simulink model "MCU_FOC_MAIN"  (R2024b)
settings: configuration reference "MODEL_CONFIG_PARENT" (kept outside this file)
settings Model: DataDictionary=MCU_FOC_MAIN_DD.sldd  EnableAccessToBaseWorkspace=off  Creator=415  LastModifiedBy=415
settings ConfigSetRef: SourceName=MODEL_CONFIG_PARENT

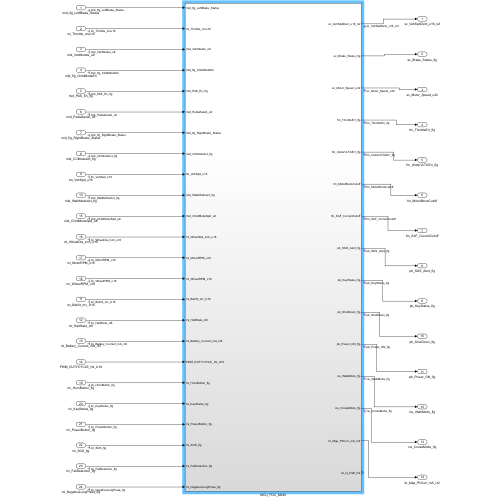
[thumbnail: Simulink's stored preview of the top-level diagram]
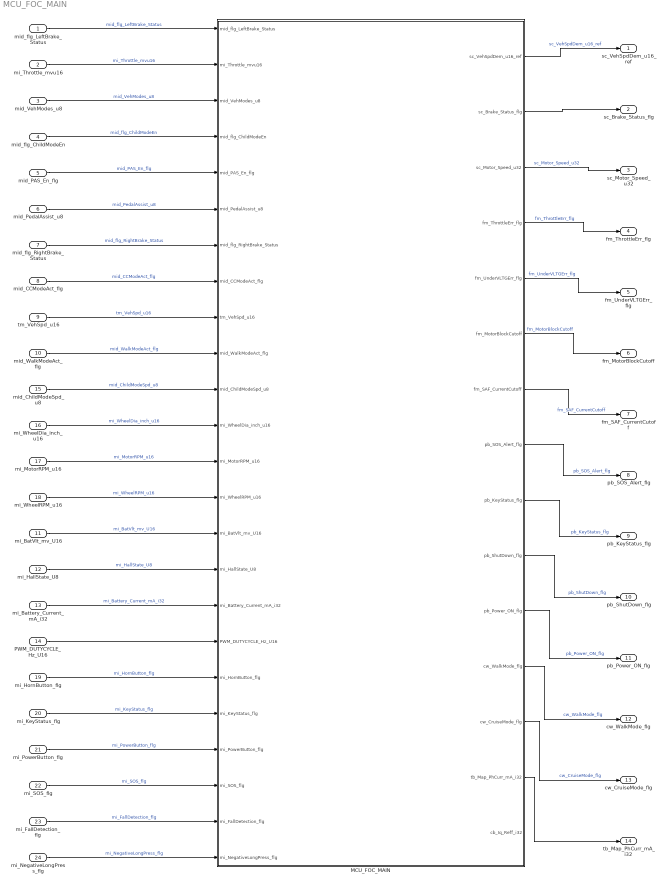
== system MCU_FOC_MAIN ==
  mid_flg_LeftBrake_Status : Inport
  mi_Throttle_mvu16 : Inport  Port=2
  mid_VehModes_u8 : Inport  Port=3
  mid_flg_ChildModeEn : Inport  Port=4
  mid_PAS_En_flg : Inport  Port=5
  mid_PedalAssist_u8 : Inport  Port=6
  mid_flg_RightBrake_Status : Inport  Port=7
  mid_CCModeAct_flg : Inport  Port=8
  tm_VehSpd_u16 : Inport  Port=9
  mid_WalkModeAct_flg : Inport  Port=10
  mi_BatVlt_mv_U16 : Inport  Port=11
  mi_HallState_U8 : Inport  Port=12
  mi_Battery_Current_mA_i32 : Inport  Port=13
  PWM_DUTYCYCLE_Hz_U16 : Inport  Port=14
  mid_ChildModeSpd_u8 : Inport  Port=15
  mi_WheelDia_inch_u16 : Inport  Port=16
  mi_MotorRPM_u16 : Inport  Port=17
  mi_WheelRPM_u16 : Inport  Port=18
  mi_HornButton_flg : Inport  Port=19
  mi_KeyStatus_flg : Inport  Port=20
  mi_PowerButton_flg : Inport  Port=21
  mi_SOS_flg : Inport  Port=22
  mi_FallDetection_flg : Inport  Port=23
  mi_NegativeLongPress_flg : Inport  Port=24
  MCU_FOC_MAIN : Subsystem
  sc_VehSpdDem_u16_ref : Outport
  sc_Brake_Status_flg : Outport  Port=2
  sc_Motor_Speed_u32 : Outport  Port=3
  fm_ThrottleErr_flg : Outport  Port=4
  fm_UnderVLTGErr_flg : Outport  Port=5
  fm_MotorBlockCutoff : Outport  Port=6
  fm_SAF_CurrentCutoff : Outport  Port=7
  pb_SOS_Alert_flg : Outport  Port=8
  pb_KeyStatus_flg : Outport  Port=9
  pb_ShutDown_flg : Outport  Port=10
  pb_Power_ON_flg : Outport  Port=11
  cw_WalkMode_flg : Outport  Port=12
  cw_CruiseMode_flg : Outport  Port=13
  tb_Map_PhCurr_mA_i32 : Outport  Port=14
  wires:
  mid_PedalAssist_u8/1 -> MCU_FOC_MAIN/6(mid_PedalAssist_u8)  "mid_PedalAssist_u8"
  mid_flg_RightBrake_Status/1 -> MCU_FOC_MAIN/7(mid_flg_RightBrake_Status)  "mid_flg_RightBrake_Status"
  mid_flg_LeftBrake_Status/1 -> MCU_FOC_MAIN/1(mid_flg_LeftBrake_Status)  "mid_flg_LeftBrake_Status"
  MCU_FOC_MAIN/13(cw_CruiseMode_flg) -> cw_CruiseMode_flg/1  "cw_CruiseMode_flg"
  mi_Throttle_mvu16/1 -> MCU_FOC_MAIN/2(mi_Throttle_mvu16)  "mi_Throttle_mvu16"
  mid_flg_ChildModeEn/1 -> MCU_FOC_MAIN/4(mid_flg_ChildModeEn)  "mid_flg_ChildModeEn"
  mi_NegativeLongPress_flg/1 -> MCU_FOC_MAIN/24(mi_NegativeLongPress_flg)  "mi_NegativeLongPress_flg"
  mid_VehModes_u8/1 -> MCU_FOC_MAIN/3(mid_VehModes_u8)  "mid_VehModes_u8"
  mi_BatVlt_mv_U16/1 -> MCU_FOC_MAIN/15(mi_BatVlt_mv_U16)  "mi_BatVlt_mv_U16"
  mid_PAS_En_flg/1 -> MCU_FOC_MAIN/5(mid_PAS_En_flg)  "mid_PAS_En_flg"
  mid_CCModeAct_flg/1 -> MCU_FOC_MAIN/8(mid_CCModeAct_flg)  "mid_CCModeAct_flg"
  MCU_FOC_MAIN/7(fm_SAF_CurrentCutoff) -> fm_SAF_CurrentCutoff/1  "fm_SAF_CurrentCutoff"
  tm_VehSpd_u16/1 -> MCU_FOC_MAIN/9(tm_VehSpd_u16)  "tm_VehSpd_u16"
  mid_WalkModeAct_flg/1 -> MCU_FOC_MAIN/10(mid_WalkModeAct_flg)  "mid_WalkModeAct_flg"
  mid_ChildModeSpd_u8/1 -> MCU_FOC_MAIN/11(mid_ChildModeSpd_u8)  "mid_ChildModeSpd_u8"
  mi_HallState_U8/1 -> MCU_FOC_MAIN/16(mi_HallState_U8)  "mi_HallState_U8"
  mi_WheelDia_inch_u16/1 -> MCU_FOC_MAIN/12(mi_WheelDia_inch_u16)  "mi_WheelDia_inch_u16"
  mi_Battery_Current_mA_i32/1 -> MCU_FOC_MAIN/17(mi_Battery_Current_mA_i32)  "mi_Battery_Current_mA_i32"
  mi_MotorRPM_u16/1 -> MCU_FOC_MAIN/13(mi_MotorRPM_u16)  "mi_MotorRPM_u16"
  MCU_FOC_MAIN/3(sc_Motor_Speed_u32) -> sc_Motor_Speed_u32/1  "sc_Motor_Speed_u32"
  PWM_DUTYCYCLE_Hz_U16/1 -> MCU_FOC_MAIN/18(PWM_DUTYCYCLE_Hz_U16)
  mi_WheelRPM_u16/1 -> MCU_FOC_MAIN/14(mi_WheelRPM_u16)  "mi_WheelRPM_u16"
  MCU_FOC_MAIN/12(cw_WalkMode_flg) -> cw_WalkMode_flg/1  "cw_WalkMode_flg"
  mi_HornButton_flg/1 -> MCU_FOC_MAIN/19(mi_HornButton_flg)  "mi_HornButton_flg"
  mi_KeyStatus_flg/1 -> MCU_FOC_MAIN/20(mi_KeyStatus_flg)  "mi_KeyStatus_flg"
  mi_PowerButton_flg/1 -> MCU_FOC_MAIN/21(mi_PowerButton_flg)  "mi_PowerButton_flg"
  mi_SOS_flg/1 -> MCU_FOC_MAIN/22(mi_SOS_flg)  "mi_SOS_flg"
  mi_FallDetection_flg/1 -> MCU_FOC_MAIN/23(mi_FallDetection_flg)  "mi_FallDetection_flg"
  MCU_FOC_MAIN/1(sc_VehSpdDem_u16_ref) -> sc_VehSpdDem_u16_ref/1  "sc_VehSpdDem_u16_ref"
  MCU_FOC_MAIN/2(sc_Brake_Status_flg) -> sc_Brake_Status_flg/1
  MCU_FOC_MAIN/4(fm_ThrottleErr_flg) -> fm_ThrottleErr_flg/1  "fm_ThrottleErr_flg"
  MCU_FOC_MAIN/8(pb_SOS_Alert_flg) -> pb_SOS_Alert_flg/1  "pb_SOS_Alert_flg"
  MCU_FOC_MAIN/5(fm_UnderVLTGErr_flg) -> fm_UnderVLTGErr_flg/1  "fm_UnderVLTGErr_flg"
  MCU_FOC_MAIN/6(fm_MotorBlockCutoff) -> fm_MotorBlockCutoff/1  "fm_MotorBlockCutoff"
  MCU_FOC_MAIN/9(pb_KeyStatus_flg) -> pb_KeyStatus_flg/1  "pb_KeyStatus_flg"
  MCU_FOC_MAIN/10(pb_ShutDown_flg) -> pb_ShutDown_flg/1  "pb_ShutDown_flg"
  MCU_FOC_MAIN/11(pb_Power_ON_flg) -> pb_Power_ON_flg/1  "pb_Power_ON_flg"
  MCU_FOC_MAIN/14(tb_Map_PhCurr_mA_i32) -> tb_Map_PhCurr_mA_i32/1

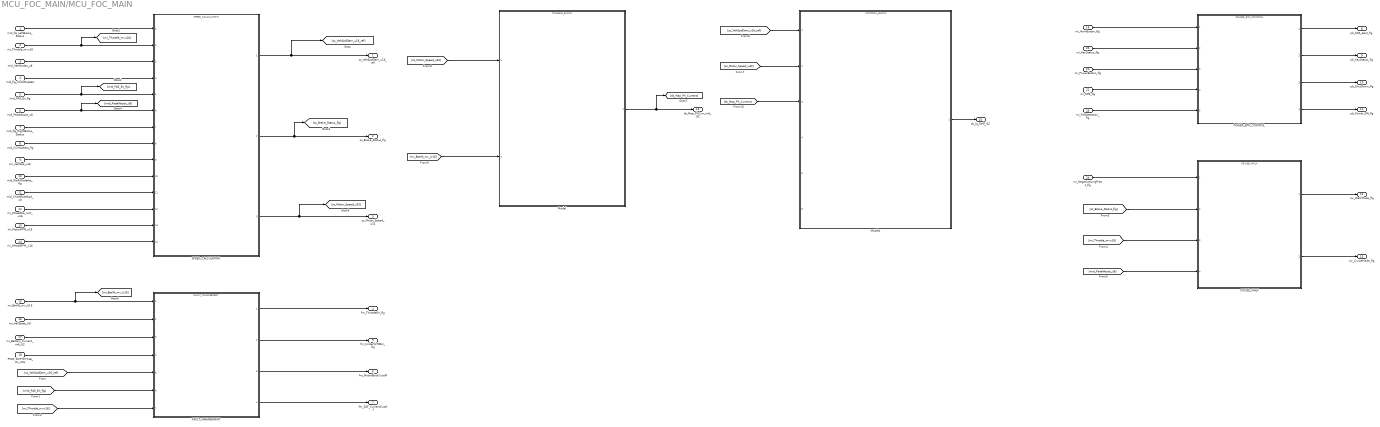
== system MCU_FOC_MAIN/MCU_FOC_MAIN ==
  mid_flg_LeftBrake_Status : Inport
  mi_Throttle_mvu16 : Inport  Port=2
  mid_VehModes_u8 : Inport  Port=3
  mid_flg_ChildModeEn : Inport  Port=4
  mid_PAS_En_flg : Inport  Port=5
  mid_PedalAssist_u8 : Inport  Port=6
  mid_flg_RightBrake_Status : Inport  Port=7
  mid_CCModeAct_flg : Inport  Port=8
  tm_VehSpd_u16 : Inport  Port=9
  mid_WalkModeAct_flg : Inport  Port=10
  mid_ChildModeSpd_u8 : Inport  Port=11
  mi_WheelDia_inch_u16 : Inport  Port=12
  mi_MotorRPM_u16 : Inport  Port=13
  mi_WheelRPM_u16 : Inport  Port=14
  mi_BatVlt_mv_U16 : Inport  Port=15
  mi_HallState_U8 : Inport  Port=16
  mi_Battery_Current_mA_i32 : Inport  Port=17
  PWM_DUTYCYCLE_Hz_U16 : Inport  Port=18
  mi_HornButton_flg : Inport  Port=19
  mi_KeyStatus_flg : Inport  Port=20
  mi_PowerButton_flg : Inport  Port=21
  mi_SOS_flg : Inport  Port=22
  mi_FallDetection_flg : Inport  Port=23
  mi_NegativeLongPress_flg : Inport  Port=24
  CRUISE_WALK : ModelReference  ModelNameDialog=CRUISE_WALK.slx  SimulationMode=Normal  ModelReferenceVersion=1.75
  FAULT_MANAGEMENT : ModelReference  ModelNameDialog=FAULT_MANAGEMENT.slx  SimulationMode=Normal  ModelReferenceVersion=1.75
  Model : ModelReference  ModelNameDialog=TUNABLE_BLOCK.slx  SimulationMode=Normal  ModelReferenceVersion=1.3
  Model4 : ModelReference  ModelNameDialog=CONTROL_BLOCK.slx  SimulationMode=Normal  ModelReferenceVersion=1.7
  POWER_BTN_CONTROL : ModelReference  ModelNameDialog=POWER_BTN_CONTROL.slx  SimulationMode=Normal  ModelReferenceVersion=1.74
  SPEED_CALCULATION : ModelReference  ModelNameDialog=SPEED_CALCULATOIN.slx  SimulationMode=Normal  ModelReferenceVersion=1.6
  sc_VehSpdDem_u16_ref : Outport
  sc_Brake_Status_flg : Outport  Port=2
  sc_Motor_Speed_u32 : Outport  Port=3
  fm_ThrottleErr_flg : Outport  Port=4
  fm_UnderVLTGErr_flg : Outport  Port=5
  fm_MotorBlockCutoff : Outport  Port=6
  fm_SAF_CurrentCutoff : Outport  Port=7
  pb_SOS_Alert_flg : Outport  Port=8
  pb_KeyStatus_flg : Outport  Port=9
  pb_ShutDown_flg : Outport  Port=10
  pb_Power_ON_flg : Outport  Port=11
  cw_WalkMode_flg : Outport  Port=12
  cw_CruiseMode_flg : Outport  Port=13
  tb_Map_PhCurr_mA_i32 : Outport  Port=14
  cb_Iq_Reff_i32 : Outport  Port=15
  wires:
  SPEED_CALCULATION/2 -> [sc_Brake_Status_flg], sc_Brake_Status_flg/1
  SPEED_CALCULATION/1 -> sc_VehSpdDem_u16_ref/1, [sc_VehSpdDem_u16_ref]
  FAULT_MANAGEMENT/3 -> fm_MotorBlockCutoff/1
  mid_PedalAssist_u8/1 -> [mid_PedalAssist_u8], SPEED_CALCULATION/6
  mid_PAS_En_flg/1 -> [mid_PAS_En_flg], SPEED_CALCULATION/5
  mid_CCModeAct_flg/1 -> SPEED_CALCULATION/8
  mi_Battery_Current_mA_i32/1 -> FAULT_MANAGEMENT/3
  [sc_VehSpdDem_u16_ref] -> FAULT_MANAGEMENT/5
  [mid_PAS_En_flg] -> FAULT_MANAGEMENT/6
  [mi_Throttle_mvu16] -> FAULT_MANAGEMENT/7
  SPEED_CALCULATION/3 -> sc_Motor_Speed_u32/1, [sc_Motor_Speed_u32]
  mid_WalkModeAct_flg/1 -> SPEED_CALCULATION/10
  mi_WheelRPM_u16/1 -> SPEED_CALCULATION/14
  FAULT_MANAGEMENT/2 -> fm_UnderVLTGErr_flg/1
  mid_flg_LeftBrake_Status/1 -> SPEED_CALCULATION/1
  mid_ChildModeSpd_u8/1 -> SPEED_CALCULATION/11
  mi_MotorRPM_u16/1 -> SPEED_CALCULATION/13
  mi_Throttle_mvu16/1 -> SPEED_CALCULATION/2, [mi_Throttle_mvu16]
  mid_VehModes_u8/1 -> SPEED_CALCULATION/3
  FAULT_MANAGEMENT/1 -> fm_ThrottleErr_flg/1
  tm_VehSpd_u16/1 -> SPEED_CALCULATION/9
  mid_flg_ChildModeEn/1 -> SPEED_CALCULATION/4
  mid_flg_RightBrake_Status/1 -> SPEED_CALCULATION/7
  mi_HallState_U8/1 -> FAULT_MANAGEMENT/2
  FAULT_MANAGEMENT/4 -> fm_SAF_CurrentCutoff/1
  mi_WheelDia_inch_u16/1 -> SPEED_CALCULATION/12
  PWM_DUTYCYCLE_Hz_U16/1 -> FAULT_MANAGEMENT/4
  mi_BatVlt_mv_U16/1 -> FAULT_MANAGEMENT/1, [mi_BatVlt_mv_U16]
  mi_SOS_flg/1 -> POWER_BTN_CONTROL/4
  mi_PowerButton_flg/1 -> POWER_BTN_CONTROL/3
  mi_FallDetection_flg/1 -> POWER_BTN_CONTROL/5
  mi_HornButton_flg/1 -> POWER_BTN_CONTROL/1
  mi_KeyStatus_flg/1 -> POWER_BTN_CONTROL/2
  POWER_BTN_CONTROL/3 -> pb_ShutDown_flg/1
  POWER_BTN_CONTROL/1 -> pb_SOS_Alert_flg/1
  POWER_BTN_CONTROL/2 -> pb_KeyStatus_flg/1
  POWER_BTN_CONTROL/4 -> pb_Power_ON_flg/1
  mi_NegativeLongPress_flg/1 -> CRUISE_WALK/1
  [mi_Throttle_mvu16] -> CRUISE_WALK/3
  [mid_PedalAssist_u8] -> CRUISE_WALK/4
  [sc_Brake_Status_flg] -> CRUISE_WALK/2
  CRUISE_WALK/1 -> cw_WalkMode_flg/1
  CRUISE_WALK/2 -> cw_CruiseMode_flg/1
  [sc_VehSpdDem_u16_ref] -> Model4/1
  [sc_Motor_Speed_u32] -> Model4/2
  Model/1 -> [tb_Map_Ph_Current], tb_Map_PhCurr_mA_i32/1
  [sc_Motor_Speed_u32] -> Model/1
  [mi_BatVlt_mv_U16] -> Model/2
  [tb_Map_Ph_Current] -> Model4/3
  Model4/1 -> cb_Iq_Reff_i32/1
